simulink library "mfcm_block_lib_v1"  (Simulink 6.1)
undefined symbols (not defined in the file or in its folder): calc_path_data, mfcm_add_phase_noise, mfcm_delay_line_depth, mfcm_dpram_format_init, mfcm_dpram_format_lsb, mfcm_dpram_format_width, mfcm_matrix_rom, mfcm_phase_noise_pacc, mfcm_phase_noise_pinc, mfcm_spectrum_roms
libraries: xbsIndex_r4 x234, mfcm_misc_lib_v1 x8, mfcm_block_lib_v1 x4, mfcm_vector_lib_v1 x3, xbsCopyrightNotice_r4 x1
(part 2 of 3)

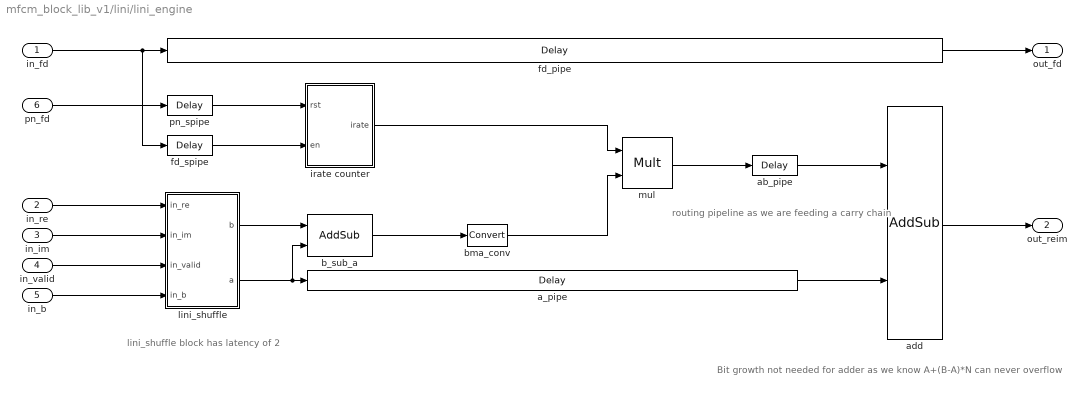
== system mfcm_block_lib_v1/lini/lini_engine ==
  note: lini_shuffle block has latency of 2
  note: Bit growth not needed for adder
      | as we know A+(B-A)*N can never overflow
  note: routing pipeline as
      | we are feeding a
      | carry chain
  in_fd : Inport  Port=1  LatchInput=off
  in_re : Inport  Port=2  LatchInput=off
  in_im : Inport  Port=3  LatchInput=off
  in_valid : Inport  Port=4  LatchInput=off
  in_b : Inport  Port=5  LatchInput=off
  pn_fd : Inport  Port=6  LatchInput=off
  a_pipe : xbsIndex_r4/Delay  en=off  latency=1+3+1  dbl_ovrd=off  reg_retiming=off  block_type=delay
      settings: infoedit="Delay line having  configurable length.<P><P>Hardware notes: A delay line is a chain, each link of which is an SRL16 followed by a flip-flop. If register retiming is enabled, the delay line is a chain of flip-flops."  xl_area=[0, 0, 0, 0, 0, 0, 0]  block_version=VER_STRING_GOES_HERE
  ab_pipe : xbsIndex_r4/Delay  en=off  latency=1  dbl_ovrd=off  reg_retiming=off  block_type=delay
      settings: infoedit="Delay line having  configurable length.<P><P>Hardware notes: A delay line is a chain, each link of which is an SRL16 followed by a flip-flop. If register retiming is enabled, the delay line is a chain of flip-flops."  xl_area=[0, 0, 0, 0, 0, 0, 0]  block_version=VER_STRING_GOES_HERE
  add : xbsIndex_r4/AddSub  mode=Addition  use_carryin=off  use_carryout=off  en=off  latency=1  precision=User Defined  arith_type="Signed  (2's comp)"  n_bits=OUT_WIDTH  bin_pt=OUT_BINPT  quantization=Truncate  overflow=Wrap  dbl_ovrd=off  use_behavioral_HDL=on  pipelined=on  use_rpm=on  block_type=addsub
      settings: xl_area=[0, 0, 0, 0, 0, 0, 0]  block_version=VER_STRING_GOES_HERE
  b_sub_a : xbsIndex_r4/AddSub  mode=Subtraction  use_carryin=off  use_carryout=off  en=off  latency=1  precision=Full  arith_type="Signed  (2's comp)"  n_bits=8  bin_pt=0  quantization=Truncate  overflow=Wrap  dbl_ovrd=off  use_behavioral_HDL=on  pipelined=on  use_rpm=on  block_type=addsub
      settings: xl_area=[0, 0, 0, 0, 0, 0, 0]  block_version=VER_STRING_GOES_HERE
  bma_conv : xbsIndex_r4/Convert  arith_type="Signed  (2's comp)"  n_bits=min(OUT_WIDTH+1,18)  bin_pt=min(OUT_WIDTH+1,18)-(OUT_WIDTH+1-OUT_BINPT)  quantization=Truncate  overflow=Wrap  latency=0  dbl_ovrd=off  pipeline=on  block_type=convert
      settings: infoedit=The input is presented at the output after quantization and overflow effects.<P><P>Hardware notes: Additional hardware is used when rounding or saturation is selected and output width is less than the input width.  xl_area=[0, 0, 0, 0, 0, 0, 0]  block_version=VER_STRING_GOES_HERE
  fd_pipe : xbsIndex_r4/Delay  en=off  latency=3+3+2  dbl_ovrd=off  reg_retiming=off  block_type=delay
      settings: infoedit="Delay line having  configurable length.<P><P>Hardware notes: A delay line is a chain, each link of which is an SRL16 followed by a flip-flop. If register retiming is enabled, the delay line is a chain of flip-flops."  xl_area=[0, 0, 0, 0, 0, 0, 0]  block_version=VER_STRING_GOES_HERE
  fd_spipe : xbsIndex_r4/Delay  en=off  latency=2  dbl_ovrd=off  reg_retiming=off  block_type=delay
      settings: infoedit="Delay line having  configurable length.<P><P>Hardware notes: A delay line is a chain, each link of which is an SRL16 followed by a flip-flop. If register retiming is enabled, the delay line is a chain of flip-flops."  xl_area=[0, 0, 0, 0, 0, 0, 0]  block_version=VER_STRING_GOES_HERE
  irate counter : Subsystem
  lini_shuffle : Subsystem
  mul : xbsIndex_r4/Mult  precision=User Defined  arith_type="Signed  (2's comp)"  n_bits=OUT_WIDTH  bin_pt=OUT_BINPT  quantization=Truncate  overflow=Wrap  en=off  latency=3  dbl_ovrd=off  use_behavioral_HDL=off  use_embedded=on  pipeline=on  use_rpm=on  placement_style=Rectangular shape  block_type=mult
      settings: infoedit=Hardware notes: To use the internal pipeline stage of the dedicated multiplier you must select 'Pipeline to Greatest Extent Possible'.  block_version=VER_STRING_GOES_HERE
  pn_spipe : xbsIndex_r4/Delay  en=off  latency=2  dbl_ovrd=off  reg_retiming=off  block_type=delay
      settings: infoedit="Delay line having  configurable length.<P><P>Hardware notes: A delay line is a chain, each link of which is an SRL16 followed by a flip-flop. If register retiming is enabled, the delay line is a chain of flip-flops."  xl_area=[0, 0, 0, 0, 0, 0, 0]  block_version=VER_STRING_GOES_HERE
  out_fd : Outport
  out_reim : Outport  Port=2
  wires:
  in_re/1 -> lini_shuffle/1(in_re)
  in_im/1 -> lini_shuffle/2(in_im)
  in_b/1 -> lini_shuffle/4(in_b)
  in_fd/1 -> fd_pipe/1, fd_spipe/1
  fd_pipe/1 -> out_fd/1
  irate counter/1(irate) -> mul/1
  b_sub_a/1 -> bma_conv/1
  lini_shuffle/2(a) -> a_pipe/1, b_sub_a/2
  add/1 -> out_reim/1
  pn_spipe/1 -> irate counter/1(rst)
  pn_fd/1 -> pn_spipe/1
  fd_spipe/1 -> irate counter/2(en)
  mul/1 -> ab_pipe/1
  a_pipe/1 -> add/2
  lini_shuffle/1(b) -> b_sub_a/1
  in_valid/1 -> lini_shuffle/3(in_valid)
  bma_conv/1 -> mul/2
  ab_pipe/1 -> add/1

== system mfcm_block_lib_v1/lini/lini_fifo ==
  note: The lini engine requires two sets of data to work over. The iDFT can generate a third.
      | There is potentially an overlap between the LINI and IDFT so we also require a fourth for synchronisation.
      | Hence the FIFO is 4*N_PATH complex coefficients deep.
  in_fd : Inport  Port=1  LatchInput=off
  in_nd : Inport  Port=2  LatchInput=off
  in_reim : Inport  Port=3  LatchInput=off
  lini_rfd : Inport  Port=4  LatchInput=off
  pn_rfd : Inport  Port=5  LatchInput=off
  Reinterpret : xbsIndex_r4/Reinterpret  force_arith_type=on  arith_type="Signed  (2's comp)"  force_bin_pt=on  bin_pt=OUT_BINPT  block_type=cast
      settings: infoedit="Changes type of samples without altering their binary representation.<P><P>Hardware notes: In hardware this block costs nothing.<P><P>Example:  Suppose the input is 6 bits wide, signed, with 2 fractional bits, and the output is forced to unsigned with 0 fractional bits.  Then an input of -2.0 (1110.00 in binary 2's complement) becomes an output of 56 (111000 in binary)."  block_version=VER_STRING_GOES_HERE
  Reinterpret1 : xbsIndex_r4/Reinterpret  force_arith_type=on  arith_type="Signed  (2's comp)"  force_bin_pt=on  bin_pt=OUT_BINPT  block_type=cast
      settings: infoedit="Changes type of samples without altering their binary representation.<P><P>Hardware notes: In hardware this block costs nothing.<P><P>Example:  Suppose the input is 6 bits wide, signed, with 2 fractional bits, and the output is forced to unsigned with 0 fractional bits.  Then an input of -2.0 (1110.00 in binary 2's complement) becomes an output of 56 (111000 in binary)."  block_version=VER_STRING_GOES_HERE
  Slice : xbsIndex_r4/Slice  nbits=OUT_WIDTH  boolean_output=off  mode=Upper Bit Location + Width  bit1=0  base1=MSB of Input  bit0=0  base0=LSB of Input  dbl_ovrd=off  block_type=slice
      settings: infoedit="Extracts a given range of bits from each input sample and presents it at the output.  The output type is ordinarily unsigned with binary point at zero, but can be Boolean when the slice is one bit wide.<P><P>Hardware notes: In hardware this block costs nothing."  block_version=VER_STRING_GOES_HERE
  Slice1 : xbsIndex_r4/Slice  nbits=OUT_WIDTH  boolean_output=off  mode=Lower Bit Location + Width  bit1=0  base1=MSB of Input  bit0=0  base0=LSB of Input  dbl_ovrd=off  block_type=slice
      settings: infoedit="Extracts a given range of bits from each input sample and presents it at the output.  The output type is ordinarily unsigned with binary point at zero, but can be Boolean when the slice is one bit wide.<P><P>Hardware notes: In hardware this block costs nothing."  block_version=VER_STRING_GOES_HERE
  dpram : mfcm_misc_lib_v1/dpram  MEM_DEPTH=2^ceil(log2(4*CHANNELS))  MEM_INIT=0  MEM_MAXDEPTH=16
  read control : Subsystem
  write control : Subsystem
  lini_fd : Outport
  out_re : Outport  Port=2
  out_im : Outport  Port=3
  valid : Outport  Port=4
  out_b : Outport  Port=5
  pn_fd : Outport  Port=6
  wires:
  read control/2(valid) -> valid/1
  write control/1(rd_fd) -> read control/1(rd_fd)
  in_fd/1 -> write control/1(in_fd)
  in_nd/1 -> write control/2(in_nd)
  in_reim/1 -> write control/3(in_reim)
  Slice/1 -> Reinterpret/1
  Reinterpret/1 -> out_re/1
  Slice1/1 -> Reinterpret1/1
  Reinterpret1/1 -> out_im/1
  lini_rfd/1 -> read control/2(lini_rfd)
  pn_rfd/1 -> read control/3(pn_rfd)
  dpram/1 -> Slice1/1, Slice/1
  read control/1(rd_add) -> dpram/1
  write control/2(wr_add) -> dpram/2
  write control/3(wr_data) -> dpram/3
  write control/4(wr_en) -> dpram/4
  read control/3(lini_fd) -> lini_fd/1
  read control/4(out_b) -> out_b/1
  read control/5(pn_fd) -> pn_fd/1

== system mfcm_block_lib_v1/lini/rate_counter ==
  en : Inport  Port=1  LatchInput=off
  Concat : xbsIndex_r4/Concat  num_inputs=2  dbl_ovrd=off  block_type=concat
      settings: block_version=VER_STRING_GOES_HERE
  Constant : xbsIndex_r4/Constant  arith_type=Boolean  const=double(RATE<=1)  n_bits=1  bin_pt=0  explicit_period=off  period=1  equ=P=C  opselect=C  inp2=PCIN>>17  opr=+  inp1=P  carry=CIN  dbl_ovrd=off  block_type=constant
      settings: block_version=VER_STRING_GOES_HERE
  Constant1 : xbsIndex_r4/Constant  arith_type=Unsigned  const=0  n_bits=max(ceil(log2(RATE)),1)  bin_pt=0  explicit_period=off  period=1  equ=P=C  opselect=C  inp2=PCIN>>17  opr=+  inp1=P  carry=CIN  dbl_ovrd=off  block_type=constant
      settings: block_version=VER_STRING_GOES_HERE
  Constant2 : xbsIndex_r4/Constant  arith_type=Unsigned  const=1  n_bits=1  bin_pt=0  explicit_period=off  period=1  equ=P=C  opselect=C  inp2=PCIN>>17  opr=+  inp1=P  carry=CIN  dbl_ovrd=off  block_type=constant
      settings: block_version=VER_STRING_GOES_HERE
  Mux : xbsIndex_r4/Mux  inputs=2  en=off  latency=0  precision=Full  arith_type="Signed  (2's comp)"  n_bits=8  bin_pt=2  quantization=Truncate  overflow=Wrap  dbl_ovrd=off  block_type=mux
      settings: xl_area=[0, 0, 0, 0, 0, 0, 0]  block_version=VER_STRING_GOES_HERE
  rate cnt : xbsIndex_r4/Counter  cnt_type=Count Limited  cnt_to=max(RATE-1,1)  operation=Up  start_count=0  cnt_by_val=1  arith_type=Unsigned  n_bits=max(ceil(log2(RATE)),1)  bin_pt=0  load_pin=off  rst=off  en=on  dbl_ovrd=off  explicit_period=off  period=1  block_type=counter
      settings: infoedit="Configurable up, down and up/down counter.<P><P>Hardware notes: Free running counters are the least expensive in hardware.  A count limited counter is implemented by combining a counter with a comparator."  xl_area=[0, 0, 0, 0, 0, 0, 0]  block_version=VER_STRING_GOES_HERE
  rfd_pipe : xbsIndex_r4/Delay  en=off  latency=1  dbl_ovrd=off  reg_retiming=off  block_type=delay
      settings: infoedit="Delay line having  configurable length.<P><P>Hardware notes: A delay line is a chain, each link of which is an SRL16 followed by a flip-flop. If register retiming is enabled, the delay line is a chain of flip-flops."  xl_area=[0, 0, 0, 0, 0, 0, 0]  block_version=VER_STRING_GOES_HERE
  rfd_relop : xbsIndex_r4/Relational  mode=a=b  en=off  latency=1  dbl_ovrd=off  block_type=relational
      settings: xl_area=[0, 0, 0, 0, 0, 0, 0]  block_version=VER_STRING_GOES_HERE
  lini_rfd : Outport
  pn_rfd : Outport  Port=2
  wires:
  en/1 -> Concat/2, rfd_pipe/1, rate cnt/1
  Mux/1 -> Concat/1
  Constant1/1 -> Mux/3
  rate cnt/1 -> Mux/2
  Constant/1 -> Mux/1
  Concat/1 -> rfd_relop/1
  Constant2/1 -> rfd_relop/2
  rfd_relop/1 -> pn_rfd/1
  rfd_pipe/1 -> lini_rfd/1

== system mfcm_block_lib_v1/phase_noise/lfsr1 ==
  note: 61 bit LFSR with 26bit leap forward. Maximal sequence with length 2^61-1.
      | gcd(2^61-1,26) is 1 (as 2^61-1 is Mersenne prime), so 26bit sequence has same period.
      | NOTE: can't use Matlab gcd for this as it only supports 56bit mantissas.
  en : Inport  Port=1  LatchInput=off
  Concat : xbsIndex_r4/Concat  num_inputs=2  dbl_ovrd=off  block_type=concat
      settings: block_version=VER_STRING_GOES_HERE
  Concat1 : xbsIndex_r4/Concat  num_inputs=2  dbl_ovrd=off  block_type=concat
      settings: block_version=VER_STRING_GOES_HERE
  Convert : xbsIndex_r4/Convert  arith_type=Unsigned  n_bits=61  bin_pt=0  quantization=Truncate  overflow=Wrap  latency=0  dbl_ovrd=off  pipeline=off  block_type=convert
      settings: infoedit=The input is presented at the output after quantization and overflow effects.<P><P>Hardware notes: Additional hardware is used when rounding or saturation is selected and output width is less than the input width.  xl_area=[0, 0, 0, 0, 0, 0, 0]  block_version=VER_STRING_GOES_HERE
  Logical : xbsIndex_r4/Logical  logical_function=XOR  inputs=4  en=off  latency=0  precision=Full  arith_type=Unsigned  n_bits=8  bin_pt=2  align_bp=on  dbl_ovrd=off  block_type=logical
      settings: xl_area=[0, 0, 0, 0, 0, 0, 0]  block_version=VER_STRING_GOES_HERE
  Register : xbsIndex_r4/Register  init=hex2dec(SEED(9:end))  rst=off  en=on  dbl_ovrd=off  block_type=register
      settings: xl_area=[0, 0, 0, 0, 0, 0, 0]  block_version=VER_STRING_GOES_HERE
  Register1 : xbsIndex_r4/Register  init=mod(hex2dec(SEED(1:8)),2^29)  rst=off  en=on  dbl_ovrd=off  block_type=register
      settings: xl_area=[0, 0, 0, 0, 0, 0, 0]  block_version=VER_STRING_GOES_HERE
  Slice : xbsIndex_r4/Slice  nbits=26  boolean_output=off  mode=Lower Bit Location + Width  bit1=0  base1=MSB of Input  bit0=0  base0=LSB of Input  dbl_ovrd=off  block_type=slice
      settings: infoedit="Extracts a given range of bits from each input sample and presents it at the output.  The output type is ordinarily unsigned with binary point at zero, but can be Boolean when the slice is one bit wide.<P><P>Hardware notes: In hardware this block costs nothing."  block_version=VER_STRING_GOES_HERE
  Slice1 : xbsIndex_r4/Slice  nbits=26  boolean_output=off  mode=Lower Bit Location + Width  bit1=0  base1=MSB of Input  bit0=1  base0=LSB of Input  dbl_ovrd=off  block_type=slice
      settings: infoedit="Extracts a given range of bits from each input sample and presents it at the output.  The output type is ordinarily unsigned with binary point at zero, but can be Boolean when the slice is one bit wide.<P><P>Hardware notes: In hardware this block costs nothing."  block_version=VER_STRING_GOES_HERE
  Slice2 : xbsIndex_r4/Slice  nbits=35  boolean_output=off  mode=Upper Bit Location + Width  bit1=0  base1=MSB of Input  bit0=1  base0=LSB of Input  dbl_ovrd=off  block_type=slice
      settings: infoedit="Extracts a given range of bits from each input sample and presents it at the output.  The output type is ordinarily unsigned with binary point at zero, but can be Boolean when the slice is one bit wide.<P><P>Hardware notes: In hardware this block costs nothing."  block_version=VER_STRING_GOES_HERE
  Slice3 : xbsIndex_r4/Slice  nbits=29  boolean_output=off  mode=Upper Bit Location + Width  bit1=0  base1=MSB of Input  bit0=1  base0=LSB of Input  dbl_ovrd=off  block_type=slice
      settings: infoedit="Extracts a given range of bits from each input sample and presents it at the output.  The output type is ordinarily unsigned with binary point at zero, but can be Boolean when the slice is one bit wide.<P><P>Hardware notes: In hardware this block costs nothing."  block_version=VER_STRING_GOES_HERE
  Slice4 : xbsIndex_r4/Slice  nbits=32  boolean_output=off  mode=Lower Bit Location + Width  bit1=0  base1=MSB of Input  bit0=0  base0=LSB of Input  dbl_ovrd=off  block_type=slice
      settings: infoedit="Extracts a given range of bits from each input sample and presents it at the output.  The output type is ordinarily unsigned with binary point at zero, but can be Boolean when the slice is one bit wide.<P><P>Hardware notes: In hardware this block costs nothing."  block_version=VER_STRING_GOES_HERE
  Slice5 : xbsIndex_r4/Slice  nbits=26  boolean_output=off  mode=Lower Bit Location + Width  bit1=0  base1=MSB of Input  bit0=15  base0=LSB of Input  dbl_ovrd=off  block_type=slice
      settings: infoedit="Extracts a given range of bits from each input sample and presents it at the output.  The output type is ordinarily unsigned with binary point at zero, but can be Boolean when the slice is one bit wide.<P><P>Hardware notes: In hardware this block costs nothing."  block_version=VER_STRING_GOES_HERE
  Slice6 : xbsIndex_r4/Slice  nbits=26  boolean_output=off  mode=Lower Bit Location + Width  bit1=0  base1=MSB of Input  bit0=16  base0=LSB of Input  dbl_ovrd=off  block_type=slice
      settings: infoedit="Extracts a given range of bits from each input sample and presents it at the output.  The output type is ordinarily unsigned with binary point at zero, but can be Boolean when the slice is one bit wide.<P><P>Hardware notes: In hardware this block costs nothing."  block_version=VER_STRING_GOES_HERE
  out_data : Outport
  wires:
  Slice6/1 -> Logical/4
  Slice5/1 -> Logical/3
  Register1/1 -> Concat/1
  Register/1 -> Concat/2
  Concat/1 -> Slice/1, Slice6/1, Slice2/1, Slice5/1, Slice1/1
  Slice/1 -> Logical/1, out_data/1
  Slice1/1 -> Logical/2
  Logical/1 -> Concat1/1
  Slice2/1 -> Concat1/2
  Slice3/1 -> Register1/1
  Slice4/1 -> Register/1
  Convert/1 -> Slice3/1, Slice4/1
  Concat1/1 -> Convert/1
  en/1 -> Register1/2, Register/2

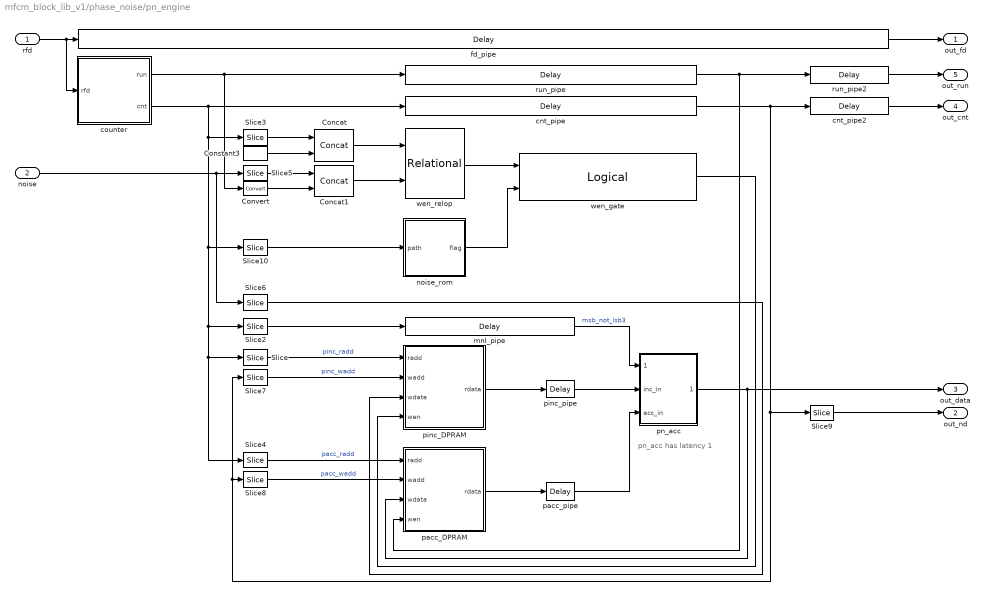
== system mfcm_block_lib_v1/phase_noise/pn_engine ==
  note: pn_acc has latency 1
  rfd : Inport  Port=1  LatchInput=off
  noise : Inport  Port=2  LatchInput=off
  Concat : xbsIndex_r4/Concat  num_inputs=2  dbl_ovrd=off  block_type=concat
      settings: block_version=VER_STRING_GOES_HERE
  Concat1 : xbsIndex_r4/Concat  num_inputs=2  dbl_ovrd=off  block_type=concat
      settings: block_version=VER_STRING_GOES_HERE
  Constant3 : xbsIndex_r4/Constant  arith_type=Unsigned  const=1  n_bits=1  bin_pt=0  explicit_period=off  period=1  equ=P=C  opselect=C  inp2=PCIN>>17  opr=+  inp1=P  carry=CIN  dbl_ovrd=off  block_type=constant
      settings: block_version=VER_STRING_GOES_HERE
  Convert : xbsIndex_r4/Convert  arith_type=Unsigned  n_bits=1  bin_pt=0  quantization=Truncate  overflow=Wrap  latency=0  dbl_ovrd=off  pipeline=off  block_type=convert
      settings: infoedit=The input is presented at the output after quantization and overflow effects.<P><P>Hardware notes: Additional hardware is used when rounding or saturation is selected and output width is less than the input width.  xl_area=[0, 0, 0, 0, 0, 0, 0]  block_version=VER_STRING_GOES_HERE
  Slice : xbsIndex_r4/Slice  nbits=ceil(log2(N_OSC*prod(size(SPEC_DATA))))  boolean_output=off  mode=Upper Bit Location + Width  bit1=0  base1=MSB of Input  bit0=0  base0=LSB of Input  dbl_ovrd=off  block_type=slice
      settings: infoedit="Extracts a given range of bits from each input sample and presents it at the output.  The output type is ordinarily unsigned with binary point at zero, but can be Boolean when the slice is one bit wide.<P><P>Hardware notes: In hardware this block costs nothing."  block_version=VER_STRING_GOES_HERE
  Slice10 : xbsIndex_r4/Slice  nbits=ceil(log2(max(prod(size(SPEC_DATA)),2)))  boolean_output=off  mode=Upper Bit Location + Width  bit1=0  base1=MSB of Input  bit0=0  base0=LSB of Input  dbl_ovrd=off  block_type=slice
      settings: infoedit="Extracts a given range of bits from each input sample and presents it at the output.  The output type is ordinarily unsigned with binary point at zero, but can be Boolean when the slice is one bit wide.<P><P>Hardware notes: In hardware this block costs nothing."  block_version=VER_STRING_GOES_HERE
  Slice2 : xbsIndex_r4/Slice  nbits=1  boolean_output=on  mode=Lower Bit Location + Width  bit1=0  base1=MSB of Input  bit0=0  base0=LSB of Input  dbl_ovrd=off  block_type=slice
      settings: infoedit="Extracts a given range of bits from each input sample and presents it at the output.  The output type is ordinarily unsigned with binary point at zero, but can be Boolean when the slice is one bit wide.<P><P>Hardware notes: In hardware this block costs nothing."  block_version=VER_STRING_GOES_HERE
  Slice3 : xbsIndex_r4/Slice  nbits=log2(N_OSC)  boolean_output=off  mode=Lower Bit Location + Width  bit1=1  base1=MSB of Input  bit0=1  base0=LSB of Input  dbl_ovrd=off  block_type=slice
      settings: infoedit="Extracts a given range of bits from each input sample and presents it at the output.  The output type is ordinarily unsigned with binary point at zero, but can be Boolean when the slice is one bit wide.<P><P>Hardware notes: In hardware this block costs nothing."  block_version=VER_STRING_GOES_HERE
  Slice4 : xbsIndex_r4/Slice  nbits=ceil(log2(2*N_OSC*prod(size(SPEC_DATA))))  boolean_output=off  mode=Upper Bit Location + Width  bit1=0  base1=MSB of Input  bit0=0  base0=LSB of Input  dbl_ovrd=off  block_type=slice
      settings: infoedit="Extracts a given range of bits from each input sample and presents it at the output.  The output type is ordinarily unsigned with binary point at zero, but can be Boolean when the slice is one bit wide.<P><P>Hardware notes: In hardware this block costs nothing."  block_version=VER_STRING_GOES_HERE
  Slice5 : xbsIndex_r4/Slice  nbits=log2(N_IDFT)  boolean_output=off  mode=Upper Bit Location + Width  bit1=0  base1=MSB of Input  bit0=0  base0=LSB of Input  dbl_ovrd=off  block_type=slice
      settings: infoedit="Extracts a given range of bits from each input sample and presents it at the output.  The output type is ordinarily unsigned with binary point at zero, but can be Boolean when the slice is one bit wide.<P><P>Hardware notes: In hardware this block costs nothing."  block_version=VER_STRING_GOES_HERE
  Slice6 : xbsIndex_r4/Slice  nbits=log2(N_IDFT)  boolean_output=off  mode=Lower Bit Location + Width  bit1=0  base1=MSB of Input  bit0=0  base0=LSB of Input  dbl_ovrd=off  block_type=slice
      settings: infoedit="Extracts a given range of bits from each input sample and presents it at the output.  The output type is ordinarily unsigned with binary point at zero, but can be Boolean when the slice is one bit wide.<P><P>Hardware notes: In hardware this block costs nothing."  block_version=VER_STRING_GOES_HERE
  Slice7 : xbsIndex_r4/Slice  nbits=ceil(log2(N_OSC*prod(size(SPEC_DATA))))  boolean_output=off  mode=Upper Bit Location + Width  bit1=0  base1=MSB of Input  bit0=0  base0=LSB of Input  dbl_ovrd=off  block_type=slice
      settings: infoedit="Extracts a given range of bits from each input sample and presents it at the output.  The output type is ordinarily unsigned with binary point at zero, but can be Boolean when the slice is one bit wide.<P><P>Hardware notes: In hardware this block costs nothing."  block_version=VER_STRING_GOES_HERE
  Slice8 : xbsIndex_r4/Slice  nbits=ceil(log2(2*N_OSC*prod(size(SPEC_DATA))))  boolean_output=off  mode=Upper Bit Location + Width  bit1=0  base1=MSB of Input  bit0=0  base0=LSB of Input  dbl_ovrd=off  block_type=slice
      settings: infoedit="Extracts a given range of bits from each input sample and presents it at the output.  The output type is ordinarily unsigned with binary point at zero, but can be Boolean when the slice is one bit wide.<P><P>Hardware notes: In hardware this block costs nothing."  block_version=VER_STRING_GOES_HERE
  Slice9 : xbsIndex_r4/Slice  nbits=1  boolean_output=on  mode=Lower Bit Location + Width  bit1=0  base1=MSB of Input  bit0=0  base0=LSB of Input  dbl_ovrd=off  block_type=slice
      settings: infoedit="Extracts a given range of bits from each input sample and presents it at the output.  The output type is ordinarily unsigned with binary point at zero, but can be Boolean when the slice is one bit wide.<P><P>Hardware notes: In hardware this block costs nothing."  block_version=VER_STRING_GOES_HERE
  cnt_pipe : xbsIndex_r4/Delay  en=off  latency=4  dbl_ovrd=off  reg_retiming=off  block_type=delay
      settings: infoedit="Delay line having  configurable length.<P><P>Hardware notes: A delay line is a chain, each link of which is an SRL16 followed by a flip-flop. If register retiming is enabled, the delay line is a chain of flip-flops."  xl_area=[0, 0, 0, 0, 0, 0, 0]  block_version=VER_STRING_GOES_HERE
  cnt_pipe2 : xbsIndex_r4/Delay  en=off  latency=1  dbl_ovrd=off  reg_retiming=off  block_type=delay
      settings: infoedit="Delay line having  configurable length.<P><P>Hardware notes: A delay line is a chain, each link of which is an SRL16 followed by a flip-flop. If register retiming is enabled, the delay line is a chain of flip-flops."  xl_area=[0, 0, 0, 0, 0, 0, 0]  block_version=VER_STRING_GOES_HERE
  counter : Subsystem
  fd_pipe : xbsIndex_r4/Delay  en=off  latency=1+4+1  dbl_ovrd=off  reg_retiming=off  block_type=delay
      settings: infoedit="Delay line having  configurable length.<P><P>Hardware notes: A delay line is a chain, each link of which is an SRL16 followed by a flip-flop. If register retiming is enabled, the delay line is a chain of flip-flops."  xl_area=[0, 0, 0, 0, 0, 0, 0]  block_version=VER_STRING_GOES_HERE
  mnl_pipe : xbsIndex_r4/Delay  en=off  latency=3  dbl_ovrd=off  reg_retiming=off  block_type=delay
      settings: infoedit="Delay line having  configurable length.<P><P>Hardware notes: A delay line is a chain, each link of which is an SRL16 followed by a flip-flop. If register retiming is enabled, the delay line is a chain of flip-flops."  xl_area=[0, 0, 0, 0, 0, 0, 0]  block_version=VER_STRING_GOES_HERE
  noise_rom : Subsystem
      mask Display:
      | disp('z^{-1}','texmode','on');
      | 
      | port_label('input',1,'path');
      | port_label('output',1,'flag');
  pacc_DPRAM : Subsystem  mask{MEM_DEPTH=2^ceil(log2(2*N_OSC*prod(size(SPEC_DATA)))), MEM_INIT=mfcm_phase_noise_pacc(SPEC_DATA,N_IDFT), OUT_WIDTH=log2(N_IDFT)}
      mask prompts: MEM_DEPTH "Memory Depth"; MEM_INIT "Initialisation Vector"; OUT_WIDTH "Output Width"
      mask Display:
      | disp('z^{-2}','texmode','on');
      | 
      | port_label('input',1,'radd');
      | port_label('input',2,'wadd');
      | port_label('input',3,'wdata');
      | port_label('input',4,'wen');
      | 
      | port_label('output',1,'rdata');
  pacc_pipe : xbsIndex_r4/Delay  en=off  latency=1  dbl_ovrd=off  reg_retiming=off  block_type=delay
      settings: infoedit="Delay line having  configurable length.<P><P>Hardware notes: A delay line is a chain, each link of which is an SRL16 followed by a flip-flop. If register retiming is enabled, the delay line is a chain of flip-flops."  xl_area=[0, 0, 0, 0, 0, 0, 0]  block_version=VER_STRING_GOES_HERE
  pinc_DPRAM : Subsystem  mask{MEM_DEPTH=2^ceil(log2(N_OSC*prod(size(SPEC_DATA)))), MEM_INIT=mfcm_phase_noise_pinc(SPEC_DATA,N_IDFT), OUT_WIDTH=log2(N_IDFT)}
      mask prompts: MEM_DEPTH "Memory Depth"; MEM_INIT "Initialisation Vector"; OUT_WIDTH "Output Width"
      mask Display:
      | disp('z^{-2}','texmode','on');
      | 
      | port_label('input',1,'radd');
      | port_label('input',2,'wadd');
      | port_label('input',3,'wdata');
      | port_label('input',4,'wen');
      | 
      | port_label('output',1,'rdata');
  pinc_pipe : xbsIndex_r4/Delay  en=off  latency=1  dbl_ovrd=off  reg_retiming=off  block_type=delay
      settings: infoedit="Delay line having  configurable length.<P><P>Hardware notes: A delay line is a chain, each link of which is an SRL16 followed by a flip-flop. If register retiming is enabled, the delay line is a chain of flip-flops."  xl_area=[0, 0, 0, 0, 0, 0, 0]  block_version=VER_STRING_GOES_HERE
  pn_acc : Subsystem
  run_pipe : xbsIndex_r4/Delay  en=off  latency=4  dbl_ovrd=off  reg_retiming=off  block_type=delay
      settings: infoedit="Delay line having  configurable length.<P><P>Hardware notes: A delay line is a chain, each link of which is an SRL16 followed by a flip-flop. If register retiming is enabled, the delay line is a chain of flip-flops."  xl_area=[0, 0, 0, 0, 0, 0, 0]  block_version=VER_STRING_GOES_HERE
  run_pipe2 : xbsIndex_r4/Delay  en=off  latency=1  dbl_ovrd=off  reg_retiming=off  block_type=delay
      settings: infoedit="Delay line having  configurable length.<P><P>Hardware notes: A delay line is a chain, each link of which is an SRL16 followed by a flip-flop. If register retiming is enabled, the delay line is a chain of flip-flops."  xl_area=[0, 0, 0, 0, 0, 0, 0]  block_version=VER_STRING_GOES_HERE
  wen_gate : xbsIndex_r4/Logical  logical_function=AND  inputs=2  en=off  latency=3  precision=Full  arith_type=Unsigned  n_bits=8  bin_pt=2  align_bp=on  dbl_ovrd=off  block_type=logical
      settings: block_version=VER_STRING_GOES_HERE
  wen_relop : xbsIndex_r4/Relational  mode=a=b  en=off  latency=1  dbl_ovrd=off  block_type=relational
      settings: xl_area=[0, 0, 0, 0, 0, 0, 0]  block_version=VER_STRING_GOES_HERE
  out_fd : Outport
  out_nd : Outport  Port=2
  out_data : Outport  Port=3
  out_cnt : Outport  Port=4
  out_run : Outport  Port=5
  wires:
  run_pipe2/1 -> out_run/1
  counter/2(cnt) -> Slice3/1, Slice/1, Slice4/1, Slice2/1, Slice10/1, cnt_pipe/1
  Slice/1 -> pinc_DPRAM/1(radd)  "pinc_radd"
  mnl_pipe/1 -> pn_acc/1(msb_not_lsb)  "msb_not_lsb3"
  Slice2/1 -> mnl_pipe/1
  Slice4/1 -> pacc_DPRAM/1(radd)  "pacc_radd"
  pn_acc/1(acc_out) -> out_data/1, pacc_DPRAM/3(wdata)
  cnt_pipe/1 -> Slice9/1, Slice7/1, Slice8/1, cnt_pipe2/1
  Slice7/1 -> pinc_DPRAM/2(wadd)  "pinc_wadd"
  Slice8/1 -> pacc_DPRAM/2(wadd)  "pacc_wadd"
  Slice9/1 -> out_nd/1
  rfd/1 -> counter/1(rfd), fd_pipe/1
  counter/1(run) -> Convert/1, run_pipe/1
  run_pipe/1 -> run_pipe2/1, pacc_DPRAM/4(wen)
  noise/1 -> Slice5/1, Slice6/1
  Constant3/1 -> Concat/2
  Slice3/1 -> Concat/1
  Slice5/1 -> Concat1/1
  Convert/1 -> Concat1/2
  Concat1/1 -> wen_relop/2
  Slice6/1 -> pinc_DPRAM/3(wdata)
  fd_pipe/1 -> out_fd/1
  Concat/1 -> wen_relop/1
  wen_gate/1 -> pinc_DPRAM/4(wen)
  cnt_pipe2/1 -> out_cnt/1
  pinc_DPRAM/1(rdata) -> pinc_pipe/1
  pacc_DPRAM/1(rdata) -> pacc_pipe/1
  pinc_pipe/1 -> pn_acc/2(inc_in)
  pacc_pipe/1 -> pn_acc/3(acc_in)
  Slice10/1 -> noise_rom/1(path)
  noise_rom/1(flag) -> wen_gate/2
  wen_relop/1 -> wen_gate/1

== system mfcm_block_lib_v1/idft/idft_engine/ST0 ==
  note: out is constant boolean 'false' with same
      | sample time as in port
  in : Inport  Port=1  LatchInput=off
  Logical : xbsIndex_r4/Logical  logical_function=XOR  inputs=2  en=off  latency=0  precision=Full  arith_type=Unsigned  n_bits=8  bin_pt=2  align_bp=on  dbl_ovrd=off  block_type=logical
      settings: xl_area=[0, 0, 0, 0, 0, 0, 0]  block_version=VER_STRING_GOES_HERE
  out : Outport
  wires:
  in/1 -> Logical/1, Logical/2
  Logical/1 -> out/1

== system mfcm_block_lib_v1/idft/idft_engine/gain ==
  note: If the map ROM is all 'zero'
      | (i.e. only one spectrum)
      | This slice should cause the map
      | ROM to optimise away
  note: This cast add a
      | '+ve' sign bit
  spec_freq : Inport  Port=1  LatchInput=off
  spec_path : Inport  Port=2  LatchInput=off
  Concat : xbsIndex_r4/Concat  num_inputs=2  dbl_ovrd=off  block_type=concat
      settings: block_version=VER_STRING_GOES_HERE
  Convert : xbsIndex_r4/Convert  arith_type="Signed  (2's comp)"  n_bits=SPEC_WIDTH+1  bin_pt=SPEC_BINPT  quantization=Truncate  overflow=Wrap  latency=0  dbl_ovrd=off  pipeline=off  block_type=convert
      settings: infoedit=The input is presented at the output after quantization and overflow effects.<P><P>Hardware notes: Additional hardware is used when rounding or saturation is selected and output width is less than the input width.  xl_area=[0, 0, 0, 0, 0, 0, 0]  block_version=VER_STRING_GOES_HERE
  Slice : xbsIndex_r4/Slice  nbits=ceil(log2(max(ROMS.map)+1))+log2(N_OSC)  boolean_output=off  mode=Lower Bit Location + Width  bit1=0  base1=MSB of Input  bit0=0  base0=LSB of Input  dbl_ovrd=off  block_type=slice
      settings: infoedit="Extracts a given range of bits from each input sample and presents it at the output.  The output type is ordinarily unsigned with binary point at zero, but can be Boolean when the slice is one bit wide.<P><P>Hardware notes: In hardware this block costs nothing."  block_version=VER_STRING_GOES_HERE
  freq_pipe : xbsIndex_r4/Delay  en=off  latency=6  dbl_ovrd=off  reg_retiming=off  block_type=delay
      settings: infoedit="Delay line having  configurable length.<P><P>Hardware notes: A delay line is a chain, each link of which is an SRL16 followed by a flip-flop. If register retiming is enabled, the delay line is a chain of flip-flops."  xl_area=[0, 0, 0, 0, 0, 0, 0]  block_version=VER_STRING_GOES_HERE
  gain_rom : xbsIndex_r4/ROM  depth=length(ROMS.gain)  initVector=ROMS.gain  distributed_mem=Block RAM  rst=off  init_reg=0  en=off  latency=2  arith_type=Unsigned  n_bits=SPEC_WIDTH  bin_pt=SPEC_BINPT  dbl_ovrd=off  use_rpm=off  block_type=sprom
      settings: xl_area=[0, 0, 0, 0, 0, 0, 0]  block_version=VER_STRING_GOES_HERE
  map_pipe : xbsIndex_r4/Delay  en=off  latency=5  dbl_ovrd=off  reg_retiming=off  block_type=delay
      settings: infoedit="Delay line having  configurable length.<P><P>Hardware notes: A delay line is a chain, each link of which is an SRL16 followed by a flip-flop. If register retiming is enabled, the delay line is a chain of flip-flops."  xl_area=[0, 0, 0, 0, 0, 0, 0]  block_version=VER_STRING_GOES_HERE
  map_rom : xbsIndex_r4/ROM  depth=2^ceil(log2(max(length(ROMS.map),2)))  initVector=ROMS.map  distributed_mem=Distributed memory  rst=off  init_reg=0  en=off  latency=1  arith_type=Unsigned  n_bits=max(ceil(log2(max(ROMS.map)+1)),1)  bin_pt=0  dbl_ovrd=off  use_rpm=off  block_type=sprom
      settings: xl_area=[0, 0, 0, 0, 0, 0, 0]  block_version=VER_STRING_GOES_HERE
  gain : Outport
  wires:
  map_rom/1 -> map_pipe/1
  map_pipe/1 -> Concat/1
  freq_pipe/1 -> Concat/2
  spec_freq/1 -> freq_pipe/1
  spec_path/1 -> map_rom/1
  Slice/1 -> gain_rom/1
  Concat/1 -> Slice/1
  Convert/1 -> gain/1
  gain_rom/1 -> Convert/1

== system mfcm_block_lib_v1/idft/idft_engine/idft_phase ==
  in_kne0 : Inport  Port=1  LatchInput=off
  in_n : Inport  Port=2  LatchInput=off
  *(N_OSC div 2) : xbsIndex_r4/Shift  shift_dir=Left  shift_bits=log2(N_OSC/2)  en=off  latency=0  precision=User Defined  arith_type=Unsigned  n_bits=log2(N_IDFT)  bin_pt=0  quantization=Truncate  overflow=Wrap  dbl_ovrd=off  block_type=shift
      settings: xl_area=[0, 0, 0, 0, 0, 0, 0]  block_version=VER_STRING_GOES_HERE
  a_mux : xbsIndex_r4/Mux  inputs=2  en=off  latency=1  precision=Full  arith_type=Unsigned  n_bits=8  bin_pt=2  quantization=Truncate  overflow=Wrap  dbl_ovrd=off  block_type=mux
      settings: block_version=VER_STRING_GOES_HERE
  b_mux : xbsIndex_r4/Mux  inputs=2  en=off  latency=1  precision=Full  arith_type=Unsigned  n_bits=8  bin_pt=2  quantization=Truncate  overflow=Wrap  dbl_ovrd=off  block_type=mux
      settings: block_version=VER_STRING_GOES_HERE
  inv : xbsIndex_r4/Inverter  en=off  latency=0  dbl_ovrd=off  block_type=inv
      settings: xl_area=[0, 0, 0, 0, 0, 0, 0]  block_version=VER_STRING_GOES_HERE
  one : xbsIndex_r4/Constant  arith_type=Unsigned  const=1  n_bits=log2(N_IDFT)  bin_pt=0  explicit_period=off  period=1  equ=P=C  opselect=C  inp2=PCIN>>17  opr=+  inp1=P  carry=CIN  dbl_ovrd=off  block_type=constant
      settings: block_version=VER_STRING_GOES_HERE
  pacc : xbsIndex_r4/AddSub  mode=Addition  use_carryin=off  use_carryout=off  en=off  latency=1  precision=User Defined  arith_type=Unsigned  n_bits=log2(N_IDFT)  bin_pt=0  quantization=Truncate  overflow=Wrap  dbl_ovrd=off  use_behavioral_HDL=on  pipelined=off  use_rpm=off  block_type=addsub
      settings: xl_area=[0, 0, 0, 0, 0, 0, 0]  block_version=VER_STRING_GOES_HERE
  out_pacc : Outport
  wires:
  b_mux/1 -> pacc/2
  a_mux/1 -> pacc/1
  inv/1 -> b_mux/2
  in_n/1 -> b_mux/3, *(N_OSC div 2)/1
  in_kne0/1 -> a_mux/1, b_mux/1
  pacc/1 -> a_mux/3, out_pacc/1
  one/1 -> a_mux/2
  *(N_OSC div 2)/1 -> inv/1

== system mfcm_block_lib_v1/lini/lini_engine/irate counter ==
  rst : Inport  Port=1  LatchInput=off
  en : Inport  Port=2  LatchInput=off
  Constant : xbsIndex_r4/Constant  arith_type=Boolean  const=double(RATE<=1)  n_bits=1  bin_pt=0  explicit_period=off  period=1  equ=P=C  opselect=C  inp2=PCIN>>17  opr=+  inp1=P  carry=CIN  dbl_ovrd=off  block_type=constant
      settings: block_version=VER_STRING_GOES_HERE
  Constant1 : xbsIndex_r4/Constant  arith_type=Signed (2's comp)  const=0  n_bits=18  bin_pt=17  explicit_period=off  period=1  equ=P=C  opselect=C  inp2=PCIN>>17  opr=+  inp1=P  carry=CIN  dbl_ovrd=off  block_type=constant
      settings: block_version=VER_STRING_GOES_HERE
  Mux1 : xbsIndex_r4/Mux  inputs=2  en=off  latency=0  precision=Full  arith_type="Signed  (2's comp)"  n_bits=8  bin_pt=2  quantization=Truncate  overflow=Wrap  dbl_ovrd=off  block_type=mux
      settings: xl_area=[0, 0, 0, 0, 0, 0, 0]  block_version=VER_STRING_GOES_HERE
  irate cnt : xbsIndex_r4/Counter  cnt_type=Free Running  cnt_to=Inf  operation=Up  start_count=0  cnt_by_val=min(1/RATE,1-2^-17)  arith_type="Signed  (2's comp)"  n_bits=18  bin_pt=17  load_pin=off  rst=on  en=on  dbl_ovrd=off  explicit_period=off  period=1  block_type=counter
      settings: infoedit="Configurable up, down and up/down counter.<P><P>Hardware notes: Free running counters are the least expensive in hardware.  A count limited counter is implemented by combining a counter with a comparator."  xl_area=[0, 0, 0, 0, 0, 0, 0]  block_version=VER_STRING_GOES_HERE
  irate : Outport
  wires:
  irate cnt/1 -> Mux1/2
  Constant1/1 -> Mux1/3
  rst/1 -> irate cnt/1
  en/1 -> irate cnt/2
  Constant/1 -> Mux1/1
  Mux1/1 -> irate/1

== system mfcm_block_lib_v1/lini/lini_engine/lini_shuffle ==
  note: Shuffle order of linear interpolation inputs for input to engine
      | Also handles valid data control
      |
      | in_re =[b0r a0r b1r a1r b2r a2r b3r a3r]
      | in_im=[b0i a0i b1i a1i b2i a2i b3i a3i]
      |
      | a=[a0r a0i a1r a1i a2r a2i a3r a3i]
      | b=[b0r b0i b1r b1i b2r b2i b3r b3i]
  in_re : Inport  Port=1  LatchInput=off
  in_im : Inport  Port=2  LatchInput=off
  in_valid : Inport  Port=3  LatchInput=off
  in_b : Inport  Port=4  LatchInput=off
  Concat : xbsIndex_r4/Concat  num_inputs=2  dbl_ovrd=off  block_type=concat
      settings: block_version=VER_STRING_GOES_HERE
  Constant1 : xbsIndex_r4/Constant  arith_type=Signed (2's comp)  const=0  n_bits=OUT_WIDTH  bin_pt=OUT_BINPT  explicit_period=off  period=1  equ=P=C  opselect=C  inp2=PCIN>>17  opr=+  inp1=P  carry=CIN  dbl_ovrd=off  block_type=constant
      settings: block_version=VER_STRING_GOES_HERE
  a_mux : xbsIndex_r4/Mux  inputs=4  en=off  latency=1  precision=Full  arith_type="Signed  (2's comp)"  n_bits=8  bin_pt=2  quantization=Truncate  overflow=Wrap  dbl_ovrd=off  block_type=mux
      settings: xl_area=[0, 0, 0, 0, 0, 0, 0]  block_version=VER_STRING_GOES_HERE
  amux_pipe0 : xbsIndex_r4/Delay  en=off  latency=1  dbl_ovrd=off  reg_retiming=off  block_type=delay
      settings: infoedit="Delay line having  configurable length.<P><P>Hardware notes: A delay line is a chain, each link of which is an SRL16 followed by a flip-flop. If register retiming is enabled, the delay line is a chain of flip-flops."  xl_area=[0, 0, 0, 0, 0, 0, 0]  block_version=VER_STRING_GOES_HERE
  b_mux : xbsIndex_r4/Mux  inputs=4  en=off  latency=1  precision=Full  arith_type="Signed  (2's comp)"  n_bits=8  bin_pt=2  quantization=Truncate  overflow=Wrap  dbl_ovrd=off  block_type=mux
      settings: xl_area=[0, 0, 0, 0, 0, 0, 0]  block_version=VER_STRING_GOES_HERE
  bmux_pipe0 : xbsIndex_r4/Delay  en=off  latency=2  dbl_ovrd=off  reg_retiming=off  block_type=delay
      settings: infoedit="Delay line having  configurable length.<P><P>Hardware notes: A delay line is a chain, each link of which is an SRL16 followed by a flip-flop. If register retiming is enabled, the delay line is a chain of flip-flops."  xl_area=[0, 0, 0, 0, 0, 0, 0]  block_version=VER_STRING_GOES_HERE
  bmux_pipe1 : xbsIndex_r4/Delay  en=off  latency=1  dbl_ovrd=off  reg_retiming=off  block_type=delay
      settings: infoedit="Delay line having  configurable length.<P><P>Hardware notes: A delay line is a chain, each link of which is an SRL16 followed by a flip-flop. If register retiming is enabled, the delay line is a chain of flip-flops."  xl_area=[0, 0, 0, 0, 0, 0, 0]  block_version=VER_STRING_GOES_HERE
  sel_pipe : xbsIndex_r4/Delay  en=off  latency=1  dbl_ovrd=off  reg_retiming=off  block_type=delay
      settings: infoedit="Delay line having  configurable length.<P><P>Hardware notes: A delay line is a chain, each link of which is an SRL16 followed by a flip-flop. If register retiming is enabled, the delay line is a chain of flip-flops."  xl_area=[0, 0, 0, 0, 0, 0, 0]  block_version=VER_STRING_GOES_HERE
  b : Outport
  a : Outport  Port=2
  wires:
  in_im/1 -> bmux_pipe0/1, amux_pipe0/1
  in_re/1 -> bmux_pipe1/1, a_mux/5
  amux_pipe0/1 -> a_mux/4
  b_mux/1 -> b/1  "b"
  a_mux/1 -> a/1  "a"
  bmux_pipe1/1 -> b_mux/5
  bmux_pipe0/1 -> b_mux/4
  in_valid/1 -> Concat/1
  in_b/1 -> Concat/2
  Concat/1 -> sel_pipe/1
  Constant1/1 -> b_mux/2, b_mux/3, a_mux/2, a_mux/3
  sel_pipe/1 -> b_mux/1, a_mux/1

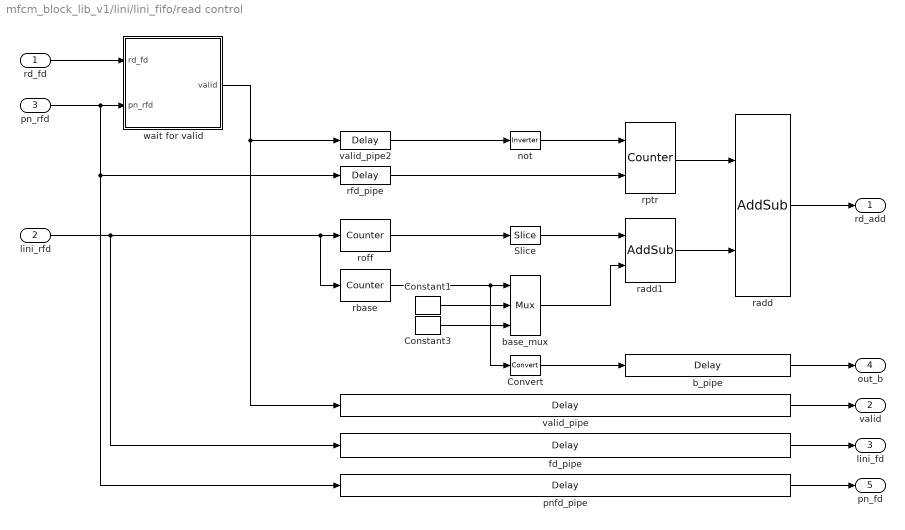
== system mfcm_block_lib_v1/lini/lini_fifo/read control ==
  rd_fd : Inport  Port=1  LatchInput=off
  lini_rfd : Inport  Port=2  LatchInput=off
  pn_rfd : Inport  Port=3  LatchInput=off
  Constant1 : xbsIndex_r4/Constant  arith_type=Unsigned  const=0  n_bits=ceil(log2(CHANNELS+1))  bin_pt=0  explicit_period=off  period=1  equ=P=C  opselect=C  inp2=PCIN>>17  opr=+  inp1=P  carry=CIN  dbl_ovrd=off  block_type=constant
      settings: block_version=VER_STRING_GOES_HERE
  Constant3 : xbsIndex_r4/Constant  arith_type=Unsigned  const=CHANNELS  n_bits=ceil(log2(CHANNELS+1))  bin_pt=0  explicit_period=off  period=1  equ=P=C  opselect=C  inp2=PCIN>>17  opr=+  inp1=P  carry=CIN  dbl_ovrd=off  block_type=constant
      settings: block_version=VER_STRING_GOES_HERE
  Convert : xbsIndex_r4/Convert  arith_type=Boolean  n_bits=8  bin_pt=6  quantization=Truncate  overflow=Wrap  latency=0  dbl_ovrd=off  pipeline=off  block_type=convert
      settings: infoedit=The input is presented at the output after quantization and overflow effects.<P><P>Hardware notes: Additional hardware is used when rounding or saturation is selected and output width is less than the input width.  xl_area=[0, 0, 0, 0, 0, 0, 0]  block_version=VER_STRING_GOES_HERE
  Slice : xbsIndex_r4/Slice  nbits=max(ceil(log2(CHANNELS)),1)  boolean_output=off  mode=Upper Bit Location + Width  bit1=0  base1=MSB of Input  bit0=0  base0=LSB of Input  dbl_ovrd=off  block_type=slice
      settings: infoedit="Extracts a given range of bits from each input sample and presents it at the output.  The output type is ordinarily unsigned with binary point at zero, but can be Boolean when the slice is one bit wide.<P><P>Hardware notes: In hardware this block costs nothing."  block_version=VER_STRING_GOES_HERE
  b_pipe : xbsIndex_r4/Delay  en=off  latency=2+2  dbl_ovrd=off  reg_retiming=off  block_type=delay
      settings: infoedit="Delay line having  configurable length.<P><P>Hardware notes: A delay line is a chain, each link of which is an SRL16 followed by a flip-flop. If register retiming is enabled, the delay line is a chain of flip-flops."  xl_area=[0, 0, 0, 0, 0, 0, 0]  block_version=VER_STRING_GOES_HERE
  base_mux : xbsIndex_r4/Mux  inputs=2  en=off  latency=0  precision=Full  arith_type="Signed  (2's comp)"  n_bits=8  bin_pt=2  quantization=Truncate  overflow=Wrap  dbl_ovrd=off  block_type=mux
      settings: xl_area=[0, 0, 0, 0, 0, 0, 0]  block_version=VER_STRING_GOES_HERE
  fd_pipe : xbsIndex_r4/Delay  en=off  latency=3+2  dbl_ovrd=off  reg_retiming=off  block_type=delay
      settings: infoedit="Delay line having  configurable length.<P><P>Hardware notes: A delay line is a chain, each link of which is an SRL16 followed by a flip-flop. If register retiming is enabled, the delay line is a chain of flip-flops."  xl_area=[0, 0, 0, 0, 0, 0, 0]  block_version=VER_STRING_GOES_HERE
  not : xbsIndex_r4/Inverter  en=off  latency=0  dbl_ovrd=off  block_type=inv
      settings: xl_area=[0, 0, 0, 0, 0, 0, 0]  block_version=VER_STRING_GOES_HERE
  pnfd_pipe : xbsIndex_r4/Delay  en=off  latency=3+2  dbl_ovrd=off  reg_retiming=off  block_type=delay
      settings: infoedit="Delay line having  configurable length.<P><P>Hardware notes: A delay line is a chain, each link of which is an SRL16 followed by a flip-flop. If register retiming is enabled, the delay line is a chain of flip-flops."  xl_area=[0, 0, 0, 0, 0, 0, 0]  block_version=VER_STRING_GOES_HERE
  radd : xbsIndex_r4/AddSub  mode=Addition  use_carryin=off  use_carryout=off  en=off  latency=1  precision=User Defined  arith_type=Unsigned  n_bits=ceil(log2(4*CHANNELS))  bin_pt=0  quantization=Truncate  overflow=Wrap  dbl_ovrd=off  use_behavioral_HDL=on  pipelined=on  use_rpm=on  block_type=addsub
      settings: xl_area=[0, 0, 0, 0, 0, 0, 0]  block_version=VER_STRING_GOES_HERE
  radd1 : xbsIndex_r4/AddSub  mode=Addition  use_carryin=off  use_carryout=off  en=off  latency=1  precision=User Defined  arith_type=Unsigned  n_bits=ceil(log2(4*CHANNELS))  bin_pt=0  quantization=Truncate  overflow=Wrap  dbl_ovrd=off  use_behavioral_HDL=on  pipelined=off  use_rpm=off  block_type=addsub
      settings: xl_area=[0, 0, 0, 0, 0, 0, 0]  block_version=VER_STRING_GOES_HERE
  rbase : xbsIndex_r4/Counter  cnt_type=Free Running  cnt_to=Inf  operation=Down  start_count=1  cnt_by_val=1  arith_type=Unsigned  n_bits=1  bin_pt=0  load_pin=off  rst=on  en=off  dbl_ovrd=off  explicit_period=off  period=1  block_type=counter
      settings: infoedit="Configurable up, down and up/down counter.<P><P>Hardware notes: Free running counters are the least expensive in hardware.  A count limited counter is implemented by combining a counter with a comparator."  xl_area=[0, 0, 0, 0, 0, 0, 0]  block_version=VER_STRING_GOES_HERE
  rfd_pipe : xbsIndex_r4/Delay  en=off  latency=1  dbl_ovrd=off  reg_retiming=off  block_type=delay
      settings: infoedit="Delay line having  configurable length.<P><P>Hardware notes: A delay line is a chain, each link of which is an SRL16 followed by a flip-flop. If register retiming is enabled, the delay line is a chain of flip-flops."  xl_area=[0, 0, 0, 0, 0, 0, 0]  block_version=VER_STRING_GOES_HERE
  roff : xbsIndex_r4/Counter  cnt_type=Count Limited  cnt_to=2*CHANNELS-1  operation=Up  start_count=0  cnt_by_val=1  arith_type=Unsigned  n_bits=max(ceil(log2(2*CHANNELS)),2)  bin_pt=0  load_pin=off  rst=on  en=off  dbl_ovrd=off  explicit_period=off  period=1  block_type=counter
      settings: infoedit="Configurable up, down and up/down counter.<P><P>Hardware notes: Free running counters are the least expensive in hardware.  A count limited counter is implemented by combining a counter with a comparator."  xl_area=[0, 0, 0, 0, 0, 0, 0]  block_version=VER_STRING_GOES_HERE
  rptr : xbsIndex_r4/Counter  cnt_type=Free Running  cnt_to=Inf  operation=Up  start_count=0  cnt_by_val=CHANNELS  arith_type=Unsigned  n_bits=ceil(log2(4*CHANNELS))  bin_pt=0  load_pin=off  rst=on  en=on  dbl_ovrd=off  explicit_period=off  period=1  block_type=counter
      settings: infoedit="Configurable up, down and up/down counter.<P><P>Hardware notes: Free running counters are the least expensive in hardware.  A count limited counter is implemented by combining a counter with a comparator."  block_version=VER_STRING_GOES_HERE
  valid_pipe : xbsIndex_r4/Delay  en=off  latency=2+2  dbl_ovrd=off  reg_retiming=off  block_type=delay
      settings: infoedit="Delay line having  configurable length.<P><P>Hardware notes: A delay line is a chain, each link of which is an SRL16 followed by a flip-flop. If register retiming is enabled, the delay line is a chain of flip-flops."  xl_area=[0, 0, 0, 0, 0, 0, 0]  block_version=VER_STRING_GOES_HERE
  valid_pipe2 : xbsIndex_r4/Delay  en=off  latency=1  dbl_ovrd=off  reg_retiming=off  block_type=delay
      settings: infoedit="Delay line having  configurable length.<P><P>Hardware notes: A delay line is a chain, each link of which is an SRL16 followed by a flip-flop. If register retiming is enabled, the delay line is a chain of flip-flops."  xl_area=[0, 0, 0, 0, 0, 0, 0]  block_version=VER_STRING_GOES_HERE
  wait for valid : Subsystem
  rd_add : Outport
  valid : Outport  Port=2
  lini_fd : Outport  Port=3
  out_b : Outport  Port=4
  pn_fd : Outport  Port=5
  wires:
  lini_rfd/1 -> roff/1, rbase/1, fd_pipe/1
  b_pipe/1 -> out_b/1
  pn_rfd/1 -> wait for valid/2(pn_rfd), pnfd_pipe/1, rfd_pipe/1
  rd_fd/1 -> wait for valid/1(rd_fd)
  wait for valid/1(valid) -> valid_pipe/1, valid_pipe2/1
  radd1/1 -> radd/2
  radd/1 -> rd_add/1
  valid_pipe/1 -> valid/1
  rptr/1 -> radd/1
  rbase/1 -> base_mux/1, Convert/1
  roff/1 -> Slice/1
  base_mux/1 -> radd1/2
  Convert/1 -> b_pipe/1
  Slice/1 -> radd1/1
  fd_pipe/1 -> lini_fd/1
  pnfd_pipe/1 -> pn_fd/1
  valid_pipe2/1 -> not/1
  rfd_pipe/1 -> rptr/2
  not/1 -> rptr/1
  Constant1/1 -> base_mux/2
  Constant3/1 -> base_mux/3
